simulink model "mdl_quadrotor_16b"  (R2016b)
settings: Solver=ode4  StartTime=0.0  StopTime=20  FixedStep=0.0001  RelTol=1e-3
undefined symbols (not defined in the file or in its folder): Acc_uDot_mPerScnd2, Acc_vDot_mPerScnd2, Acc_wDot_mPerScnd2, Ag_phi_rad, Ag_psi_rad, Ag_theta_rad, AgVel_p_radPerScnd, AgVel_q_radPerScnd, AgVel_r_radPerScnd, Par_mdlQuad, Pos_x_mtr, Pos_y_mtr, Pos_z_mtr, V_u_mtrPerScnd, V_v_mtrPerScnd, V_w_mtrPerScnd
libraries: vrlib x2
settings Model: Creator=Nu  LastModifiedBy=Nu
settings ModelReferenceCC: ModelReferenceNumInstancesAllowed=Single

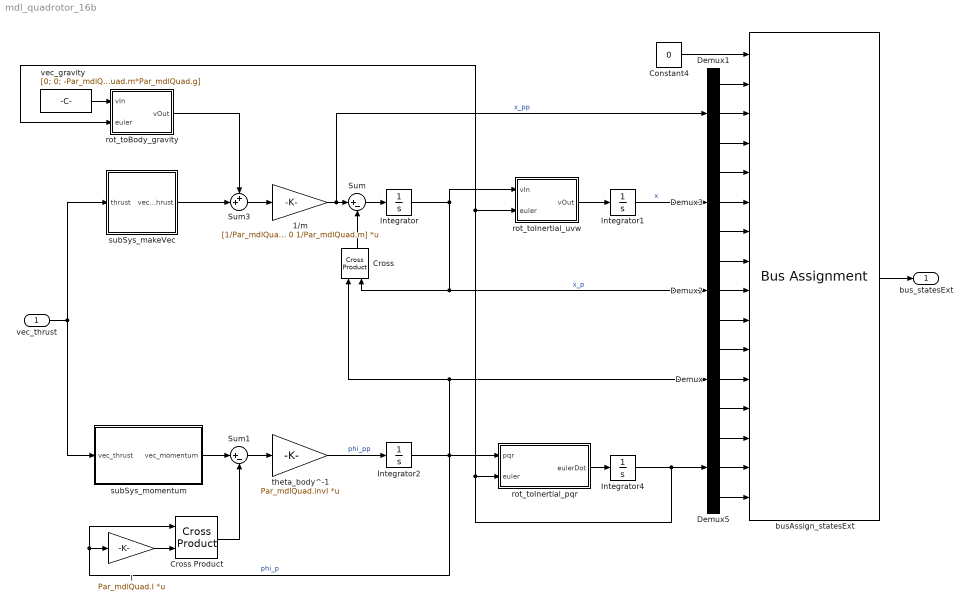
== system mdl_quadrotor_16b ==
  vec_thrust : Inport  PortDimensions=4
  1/m : Gain  Gain=[1/Par_mdlQuad.m 0 0; 0 1/Par_mdlQuad.m 0; 0 0 1/Par_mdlQuad.m]  Multiplication=Matrix(K*u)
  Constant4 : Constant  Value=0  OutDataTypeStr=Bus: mdl_statesExt
  Cross : vrlib/Utilities/Cross Product
  Cross Product : vrlib/Utilities/Cross Product
  Demux{,1..3,5} (5 alike) : Demux  Outputs=3
  I : Gain  Gain=Par_mdlQuad.I  Multiplication=Matrix(K*u)
  Integrator{,1..2,4} (4 alike) : Integrator
  Sum : Sum  Inputs=|+-
  Sum1 : Sum  Inputs=|+-
  Sum3 : Sum  Inputs=++|
  busAssign_statesExt : BusAssignment  AssignedSignals=Acc_uDot_mPerScnd2,Acc_vDot_mPerScnd2,Acc_wDot_mPerScnd2,Pos_x_mtr,Pos_y_mtr,Pos_z_mtr,V_u_mtrPerScnd,V_v_mtrPerScnd,V_w_mtrPerScnd,AgVel_p_radPerScnd,AgVel_q_radPerScnd,AgVel_r_radPerScnd,Ag_phi_rad,Ag_theta_rad,Ag_psi_rad
  rot_toBody_gravity : MATLAB Function  TreatAsAtomicUnit=on
  rot_toInertial_pqr : MATLAB Function  TreatAsAtomicUnit=on
  rot_toInertial_uvw : MATLAB Function  TreatAsAtomicUnit=on
  subSys_makeVec : Subsystem
  subSys_momentum : Subsystem
  theta_body^-1 : Gain  Gain=Par_mdlQuad.invI  Multiplication=Matrix(K*u)
  vec_gravity : Constant  Value=[0; 0; -Par_mdlQuad.m*Par_mdlQuad.g]
  "bus_statesExt " : Outport  OutDataTypeStr=Bus: mdl_statesExt
  wires:
  busAssign_statesExt/1 -> "bus_statesExt "/1
  subSys_makeVec/1(vec_thrust) -> Sum3/2
  subSys_momentum/1(vec_momentum) -> Sum1/1
  vec_thrust/1 -> subSys_makeVec/1(thrust), subSys_momentum/1(vec_thrust)
  Demux5/3 -> busAssign_statesExt/16
  Demux5/1 -> busAssign_statesExt/14
  Demux5/2 -> busAssign_statesExt/15
  Demux3/3 -> busAssign_statesExt/7
  Demux3/2 -> busAssign_statesExt/6
  Demux3/1 -> busAssign_statesExt/5
  Demux/3 -> busAssign_statesExt/13
  Demux/1 -> busAssign_statesExt/11
  Demux/2 -> busAssign_statesExt/12
  Constant4/1 -> busAssign_statesExt/1
  Demux2/3 -> busAssign_statesExt/10
  Demux2/2 -> busAssign_statesExt/9
  Demux2/1 -> busAssign_statesExt/8
  Demux1/3 -> busAssign_statesExt/4
  Demux1/2 -> busAssign_statesExt/3
  Demux1/1 -> busAssign_statesExt/2
  Cross Product/1 -> Sum1/2
  I/1 -> Cross Product/2
  Sum1/1 -> theta_body^-1/1
  theta_body^-1/1 -> Integrator2/1  "phi_pp"
  Integrator2/1 -> rot_toInertial_pqr/1(pqr), Demux/1, Cross/1, Cross Product/1, I/1  "phi_p"
  Integrator1/1 -> Demux3/1  "x"
  Integrator/1 -> rot_toInertial_uvw/1(vIn), Cross/2, Demux2/1  "x_p"
  1/m/1 -> Demux1/1, Sum/1  "x_pp"
  Sum3/1 -> 1/m/1
  rot_toInertial_pqr/1(eulerDot) -> Integrator4/1
  rot_toBody_gravity/1(vOut) -> Sum3/1
  vec_gravity/1 -> rot_toBody_gravity/1(vIn)
  Cross/1 -> Sum/2
  rot_toInertial_uvw/1(vOut) -> Integrator1/1
  Integrator4/1 -> rot_toBody_gravity/2(euler), rot_toInertial_uvw/2(euler), rot_toInertial_pqr/2(euler), Demux5/1
  Sum/1 -> Integrator/1

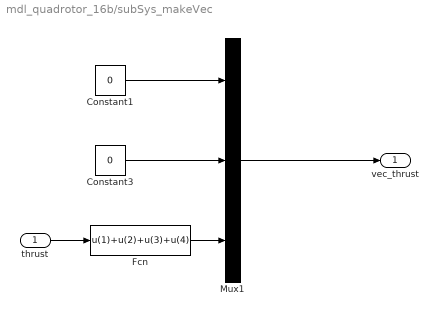
== system mdl_quadrotor_16b/subSys_makeVec ==
  thrust : Inport
  Constant1 : Constant  Value=0
  Constant3 : Constant  Value=0
  Fcn : Fcn  Expr=u(1)+u(2)+u(3)+u(4)
  Mux1 : Mux  Inputs=3
  vec_thrust : Outport
  wires:
  Fcn/1 -> Mux1/3
  Constant1/1 -> Mux1/1
  Mux1/1 -> vec_thrust/1
  Constant3/1 -> Mux1/2
  thrust/1 -> Fcn/1

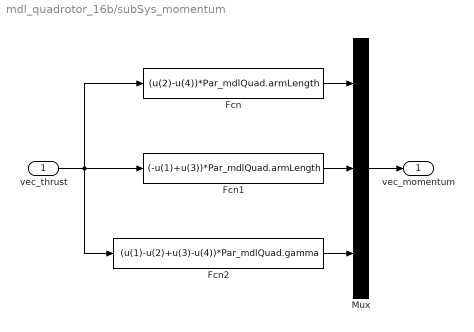
== system mdl_quadrotor_16b/subSys_momentum ==
  vec_thrust : Inport
  Fcn : Fcn  Expr=(u(2)-u(4))*Par_mdlQuad.armLength
  Fcn1 : Fcn  Expr=(-u(1)+u(3))*Par_mdlQuad.armLength
  Fcn2 : Fcn  Expr=(u(1)-u(2)+u(3)-u(4))*Par_mdlQuad.gamma
  Mux : Mux  Inputs=3
  vec_momentum : Outport
  wires:
  Fcn/1 -> Mux/1
  Fcn1/1 -> Mux/2
  Fcn2/1 -> Mux/3
  Mux/1 -> vec_momentum/1
  vec_thrust/1 -> Fcn/1, Fcn1/1, Fcn2/1

== matlab function mdl_quadrotor_16b/rot_toInertial_uvw ==
  data: vIn input; euler input; vOut output
function vOut = fcn(vIn, euler)

vOut    = rot_euler(vIn, euler, 'to-inertial-frame');

== matlab function mdl_quadrotor_16b/rot_toInertial_pqr ==
  data: pqr input; euler input; eulerDot output
function eulerDot = fcn(pqr, euler)

eulerDot = rot_karman(pqr, euler, 'to-inertial-frame');

== matlab function mdl_quadrotor_16b/rot_toBody_gravity ==
  data: vIn input; euler input; vOut output
function vOut = fcn(vIn, euler)

vOut    = rot_euler(vIn, euler, 'to-body-frame');
